simulink model "sldemo_VariableTransportDelay_org"  (Simulink 10.0)
settings: Solver=ode45  StartTime=0.0  StopTime=10.0  MaxStep=0.01  RelTol=1e-3  EnableMultiTasking=on
libraries: simulink x2
Description:
  | Vertical displacement of the wheels of a one dimensional car
  | 
  |  A car is running along a road with speed v(t). A sensor is installed
  |  at the front wheel to measure the vertical displacement Hi(t) of the
  |  the front wheel caused by the road profile. If the wheels and road
  |  never lose contact, then the vertifical displacement of the rear wheel,
  |  Ho(t), can be seen as a variable transport delay of Hi(t), which is
  |  determined by the length L between the two wheels and the speed v(t).
settings Model: Creator=The MathWorks, Inc.  LastModifiedBy=bhisma  ExtModeAutoUpdateStatusClock=off
settings DataIOCC: SaveState=on  ReturnWorkspaceOutputs=on
settings OptimizationCC: ExpressionDepthLimit=2147483647  InitFltsAndDblsToZero=on
settings DebuggingCC: SaveWithParameterizedLinksMsg=none  SignalResolutionControl=TryResolveAllWithWarning  SolverPrmCheckMsg=warning  MultiTaskDSMMsg=warning  MultiTaskCondExecSysMsg=none  SigSpecEnsureSampleTimeMsg=none  FcnCallInpInsideContextMsg=warning  StateNameClashWarn=warning
settings GRTTargetCC: TargetFcnLib=ansi_tfl_tmw.mat  GeneratePreprocessorConditionals=Disable all
settings ConfigComp: CovExternalEMLEnable=off

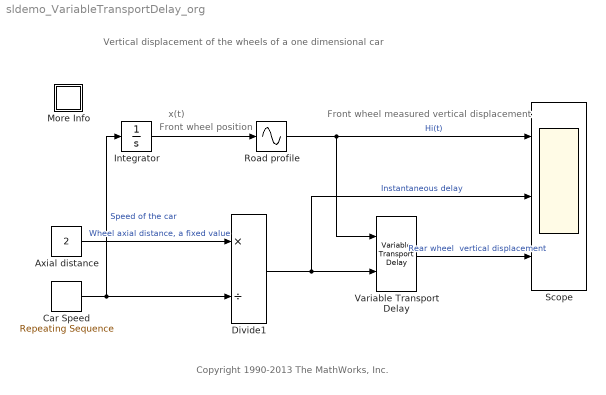
== system sldemo_VariableTransportDelay_org ==
  note: Vertical displacement of the wheels of a one dimensional car
  note: Copyright 1990-2013 The MathWorks, Inc.
  note: Front wheel measured vertical displacement
  note: x(t)
  note: Front wheel position
  Axial distance : Constant  Value=2
  Car Speed : simulink/Sources/Repeating Sequence  rep_seq_t=[0 2 4]  rep_seq_y=[1 15 1]
  Divide1 : Product  Inputs=*/
  Integrator : Integrator
  More Info : Subsystem
      settings: OpenFcn=showExample('simulink_general/sldemo_VariableTransportDelayExample')
      mask Display: disp('?')
  Road profile : Sin  TimeSource=Use external signal  Amplitude=2  Bias=2  SampleTime=0
  Scope : Scope  NumInputPorts=3
  Variable Transport Delay : VariableTransportDelay  VariableDelayType=Variable transport delay  MaximumDelay=1000  MaximumPoints=102400
  wires:
  Axial distance/1 -> Divide1/1  "Wheel axial distance, a fixed value"
  Divide1/1 -> Variable Transport Delay/2, Scope/2  "Instantaneous delay"
  Variable Transport Delay/1 -> Scope/3  "Rear wheel  vertical displacement"
  Car Speed/1 -> Divide1/2, Integrator/1  "Speed of the car"
  Road profile/1 -> Variable Transport Delay/1, Scope/1  "Hi(t)"
  Integrator/1 -> Road profile/1

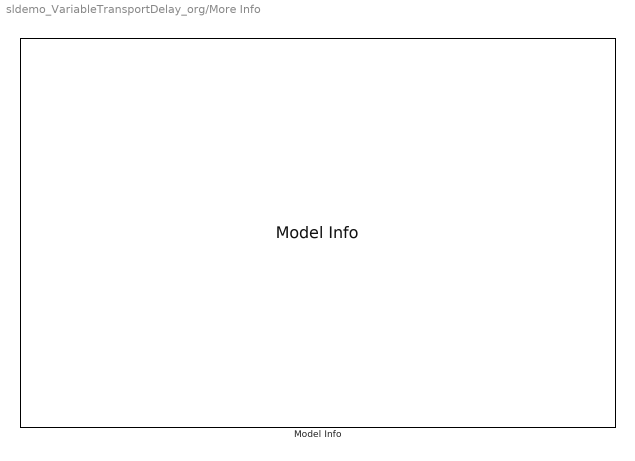
== system sldemo_VariableTransportDelay_org/More Info ==
  Model Info : simulink/Model-Wide Utilities/Model Info  Frame=on  DisplayStringWithTags=Model Info  HorizontalTextAlignment=Left  LeftAlignmentValue=0.02
